simulink model "controller1"  (Simulink 7.6)
settings: Solver=ode45  StartTime=0.0  StopTime=te  MinStep=1e-9  RelTol=1e-3
undefined symbols (not defined in the file): K, traj
libraries: commnoisgen2 x4, simulink_extras x1
settings Model: Creator=tarik  LastModifiedBy=tarik

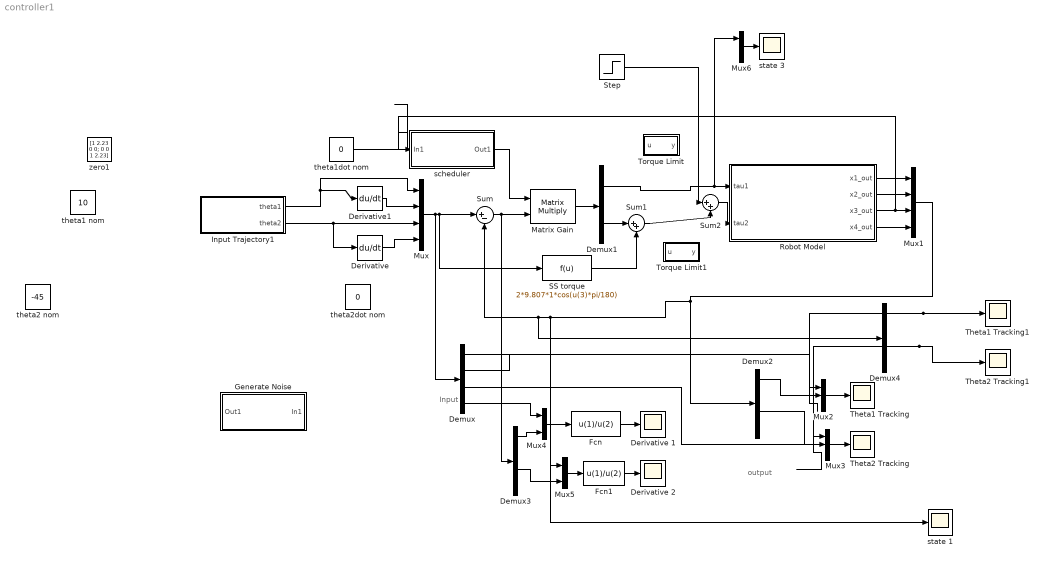
== system controller1 ==
  note: Input
  note: output
  Demux{,2..4} (4 alike) : Demux
  Demux1 : Demux  Outputs=2
  Derivative : Derivative
  Derivative 1 : Scope
      settings: TimeRange=0.09  YMin=0  YMax=70  SaveName=ScopeData3
  Derivative 2 : Scope
      settings: TimeRange=0.09  YMin=0  YMax=70  SaveName=ScopeData4
  Derivative1 : Derivative
  Fcn : Fcn  Expr=u(1)/u(2)
  Fcn1 : Fcn  Expr=u(1)/u(2)
  Generate Noise : Subsystem
  Input Trajectory1 : Subsystem
  Matrix Gain : Product  Multiplication=Matrix(*)
  Mux : Mux
  Mux1 : Mux
  Mux2 : Mux  Inputs=3
  Mux3 : Mux  Inputs=3
  Mux4 : Mux  Inputs=2
  Mux5 : Mux  Inputs=2
  Mux6 : Mux  Inputs=2
  Robot Model : Subsystem
  SS torque : Fcn  Expr=2*9.807*1*cos(u(3)*pi/180)
  Step : Step  Time=3  After=0  SampleTime=0
  Sum : Sum  Inputs=|+-
  Sum1 : Sum  Inputs=|++
  Sum2 : Sum  Inputs=|++
  Theta1 Tracking : Scope
      settings: TimeRange=0.09  YMin=-120  YMax=30
  Theta1 Tracking1 : Scope
      settings: TimeRange=0.09  YMin=-171  YMax=-163.5  SaveName=ScopeData5
  Theta2 Tracking : Scope
      settings: TimeRange=0.09  YMin=-90  YMax=-25
  Theta2 Tracking1 : Scope
      settings: TimeRange=0.09  YMin=-90  YMax=-25  SaveName=ScopeData6
  Torque Limit : Stateflow chart  TreatAsAtomicUnit=on
  Torque Limit1 : Stateflow chart  TreatAsAtomicUnit=on
  scheduler : Subsystem
  state 1 : Scope
      settings: TimeRange=0.09  YMin=-180  YMax=30  SaveName=ScopeData7
  state 3 : Scope
      settings: TimeRange=0.09  YMin=-80  YMax=80  SaveName=ScopeData2
  theta1 nom : Constant  Value=10
  theta1dot nom : Constant  Value=0
  theta2 nom : Constant  Value=-45
  theta2dot nom : Constant  Value=0
  zero1 : Constant  Value=[1 2.23 0 0; 0 0 1 2.23]
  wires:
  Mux/1 -> Demux/1, Sum/1, SS torque/1
  Robot Model/1(x1_out) -> Mux1/1
  Robot Model/2(x2_out) -> Mux1/2
  Robot Model/4(x4_out) -> Mux1/4
  Mux1/1 -> Demux2/1, Sum/2, Demux4/1, state 1/1
  Sum1/1 -> Sum2/2
  SS torque/1 -> Sum1/2
  Matrix Gain/1 -> Demux1/1
  Demux1/2 -> Sum1/1
  Sum/1 -> Matrix Gain/2, Demux3/1
  Demux1/1 -> Robot Model/1(tau1), Mux6/1
  Input Trajectory1/1(theta1) -> Mux/1, Derivative1/1
  Demux2/1 -> Mux2/2
  Mux2/1 -> Theta1 Tracking/1
  Mux3/1 -> Theta2 Tracking/1
  scheduler/1(Out1) -> Matrix Gain/1
  Input Trajectory1/2(theta2) -> Mux/3, Derivative/1
  Demux/3 -> Mux3/1
  Demux2/3 -> Mux3/2
  Derivative1/1 -> Mux/2
  Derivative/1 -> Mux/4
  Mux4/1 -> Fcn/1
  Demux/2 -> Mux5/1
  Demux/4 -> Mux4/1
  Demux3/1 -> Mux4/2
  Demux3/3 -> Mux5/2
  Mux5/1 -> Fcn1/1
  Fcn1/1 -> Derivative 2/1
  Fcn/1 -> Derivative 1/1
  Demux/1 -> Mux2/1
  Robot Model/3(x3_out) -> Mux1/3
  Mux6/1 -> state 3/1
  Sum2/1 -> Robot Model/2(tau2)
  Step/1 -> Sum2/1
  Demux4/1 -> Theta1 Tracking1/1
  Demux4/3 -> Theta2 Tracking1/1
  theta1dot nom/1 -> scheduler/1(In1)

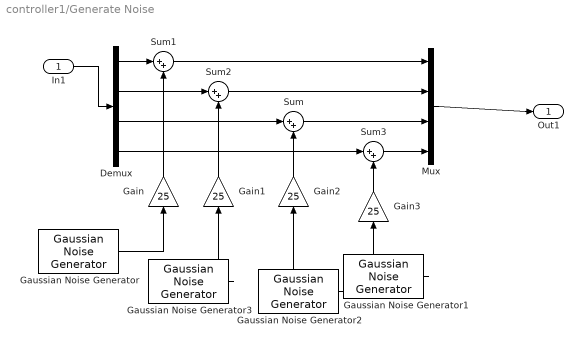
== system controller1/Generate Noise ==
  In1 : Inport
  Demux : Demux
  Gain{,1..3} (4 alike) : Gain  Gain=25
  Gaussian Noise Generator : commnoisgen2/Gaussian Noise Generator  SystemSampleTime=-1  m=0  d=1  s=41  Ts=0.1  frameBased=off  sampPerFrame=1  orient=off  outDataType=double
  Gaussian Noise Generator1 : commnoisgen2/Gaussian Noise Generator  SystemSampleTime=-1  m=0  d=1  s=41  Ts=0.1  frameBased=off  sampPerFrame=1  orient=off  outDataType=double
  Gaussian Noise Generator2 : commnoisgen2/Gaussian Noise Generator  SystemSampleTime=-1  m=0  d=1  s=41  Ts=.1  frameBased=off  sampPerFrame=1  orient=off  outDataType=double
  Gaussian Noise Generator3 : commnoisgen2/Gaussian Noise Generator  SystemSampleTime=-1  m=0  d=1  s=41  Ts=0.1  frameBased=off  sampPerFrame=1  orient=off  outDataType=double
  Mux : Mux
  Sum{,1..3} (4 alike) : Sum  Inputs=|++
  Out1 : Outport
  wires:
  In1/1 -> Demux/1
  Mux/1 -> Out1/1
  Demux/1 -> Sum1/1
  Demux/2 -> Sum2/1
  Demux/3 -> Sum/1
  Demux/4 -> Sum3/1
  Gaussian Noise Generator1/1 -> Gain3/1
  Gaussian Noise Generator2/1 -> Gain2/1
  Gaussian Noise Generator3/1 -> Gain1/1
  Gaussian Noise Generator/1 -> Gain/1
  Sum1/1 -> Mux/1
  Sum2/1 -> Mux/2
  Sum/1 -> Mux/3
  Sum3/1 -> Mux/4
  Gain/1 -> Sum1/2
  Gain1/1 -> Sum2/2
  Gain2/1 -> Sum/2
  Gain3/1 -> Sum3/2

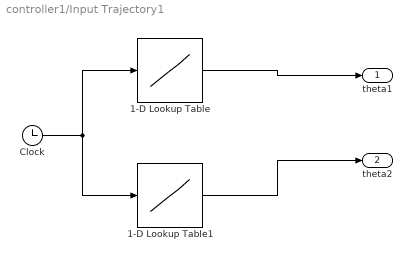
== system controller1/Input Trajectory1 ==
  1-D Lookup Table : Lookup_n-D  NumberOfTableDimensions=1  BreakpointsForDimension1=t  Table=traj(1,:)  RndMeth=Simplest  InputSameDT=on
  1-D Lookup Table1 : Lookup_n-D  NumberOfTableDimensions=1  BreakpointsForDimension1=t  Table=traj(2,:)  RndMeth=Simplest  InputSameDT=on
  Clock : Clock
      settings: Decimation=10
  theta1 : Outport
  theta2 : Outport  Port=2
  wires:
  Clock/1 -> 1-D Lookup Table/1, 1-D Lookup Table1/1
  1-D Lookup Table/1 -> theta1/1
  1-D Lookup Table1/1 -> theta2/1

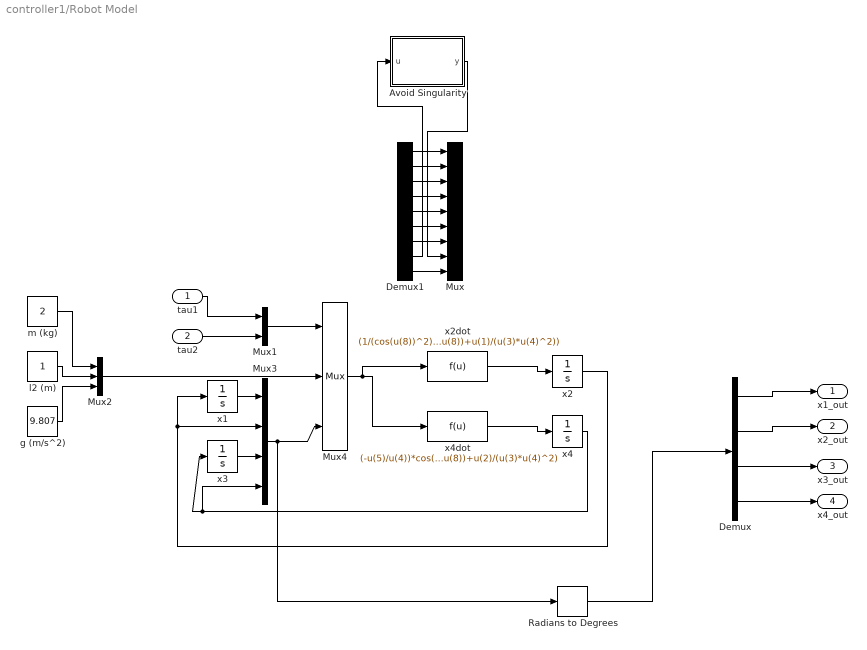
== system controller1/Robot Model ==
  tau1 : Inport
  tau2 : Inport  Port=2
  Avoid Singularity : Stateflow chart  TreatAsAtomicUnit=on
  Demux : Demux
  Demux1 : Demux  Outputs=9
  Mux : Mux  Inputs=9
  Mux1 : Mux  Inputs=2
  Mux2 : Mux  Inputs=3
  Mux3 : Mux
  Mux4 : Mux  Description=|  Inputs=3
      | u(1:2) are u1 and u2   
      | u(3:5) are m, l2, and g
      | u(6:9) are x1 x2 x3 x4
  Radians to Degrees : simulink_extras/Transformations/Radians to Degrees  SystemSampleTime=-1
  g (m/s^2) : Constant  Value=9.807
  l2 (m) : Constant
  m (kg) : Constant  Value=2
  x1 : Integrator
  x2 : Integrator
  x2dot : Fcn  Expr=(1/(cos(u(8))^2))*(u(7)*u(9)*sin(2*u(8))+u(1)/(u(3)*u(4)^2))
  x3 : Integrator  InitialCondition=0*pi/180
  x4 : Integrator
  x4dot : Fcn  Expr=(-u(5)/u(4))*cos(u(8))-(u(7)/2)*sin(2*u(8))+u(2)/(u(3)*u(4)^2)
  x1_out : Outport
  x2_out : Outport  Port=2
  x3_out : Outport  Port=3
  x4_out : Outport  Port=4
  wires:
  m (kg)/1 -> Mux2/1
  l2 (m)/1 -> Mux2/2
  g (m/s^2)/1 -> Mux2/3
  x2dot/1 -> x2/1
  x4dot/1 -> x4/1
  Mux3/1 -> Mux4/3, Radians to Degrees/1
  Mux1/1 -> Mux4/1
  x3/1 -> Mux3/3
  x4/1 -> Mux3/4, x3/1
  Mux4/1 -> x4dot/1, x2dot/1
  x2/1 -> Mux3/2, x1/1
  x1/1 -> Mux3/1
  Demux/1 -> x1_out/1
  Demux/2 -> x2_out/1
  Demux/3 -> x3_out/1
  Demux/4 -> x4_out/1
  Radians to Degrees/1 -> Demux/1
  tau1/1 -> Mux1/1
  tau2/1 -> Mux1/2
  Mux2/1 -> Mux4/2
  Demux1/1 -> Mux/1
  Demux1/2 -> Mux/2
  Demux1/3 -> Mux/3
  Demux1/4 -> Mux/4
  Demux1/5 -> Mux/5
  Demux1/6 -> Mux/6
  Demux1/7 -> Mux/7
  Demux1/9 -> Mux/9
  Demux1/8 -> Avoid Singularity/1(u)
  Avoid Singularity/1(y) -> Mux/8

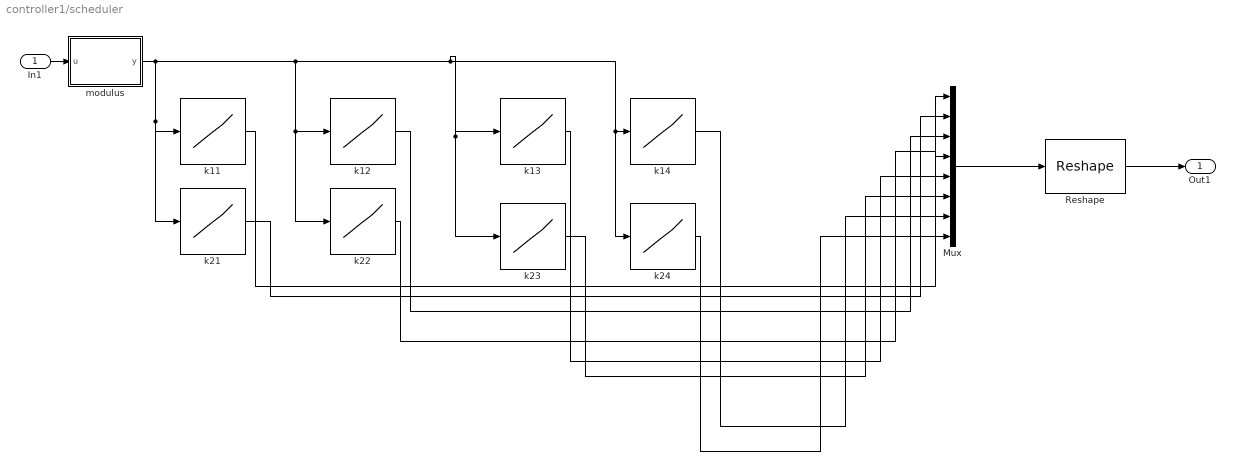
== system controller1/scheduler ==
  In1 : Inport
  Mux : Mux  Inputs=8
  Reshape : Reshape  OutputDimensionality=Customize  OutputDimensions=[2,4]
  k11 : Lookup_n-D  NumberOfTableDimensions=1  BreakpointsForDimension1=[-90:5:90]  Table=K(1,:)  RndMeth=Simplest  InputSameDT=on
  k12 : Lookup_n-D  NumberOfTableDimensions=1  BreakpointsForDimension1=[-90:5:90]  Table=K(3,:)  RndMeth=Simplest  InputSameDT=on
  k13 : Lookup_n-D  NumberOfTableDimensions=1  BreakpointsForDimension1=[-90:5:90]  Table=K(5,:)  RndMeth=Simplest  InputSameDT=on
  k14 : Lookup_n-D  NumberOfTableDimensions=1  BreakpointsForDimension1=[-90:5:90]  Table=K(7,:)  RndMeth=Simplest  InputSameDT=on
  k21 : Lookup_n-D  NumberOfTableDimensions=1  BreakpointsForDimension1=[-90:5:90]  Table=K(2,:)  RndMeth=Simplest  InputSameDT=on
  k22 : Lookup_n-D  NumberOfTableDimensions=1  BreakpointsForDimension1=[-90:5:90]  Table=K(4,:)  RndMeth=Simplest  InputSameDT=on
  k23 : Lookup_n-D  NumberOfTableDimensions=1  BreakpointsForDimension1=[-90:5:90]  Table=K(6,:)  RndMeth=Simplest  InputSameDT=on
  k24 : Lookup_n-D  NumberOfTableDimensions=1  BreakpointsForDimension1=[-90:5:90]  Table=K(8,:)  RndMeth=Simplest  InputSameDT=on
  modulus : Stateflow chart  TreatAsAtomicUnit=on
  Out1 : Outport
  wires:
  In1/1 -> modulus/1(u)
  Reshape/1 -> Out1/1
  Mux/1 -> Reshape/1
  k11/1 -> Mux/1
  k21/1 -> Mux/2
  k12/1 -> Mux/3
  k22/1 -> Mux/4
  k13/1 -> Mux/5
  k23/1 -> Mux/6
  k14/1 -> Mux/7
  k24/1 -> Mux/8
  modulus/1(y) -> k24/1, k14/1, k23/1, k13/1, k22/1, k12/1, k21/1, k11/1

== matlab function Robot Model/Avoid Singularity ==
  data: u input double; y output double
function y = fcn(u)
    th = 0.1;
    if(abs(u) > 90-th && abs(u) < 90)
        u = (90-th)*abs(u)/u;
    elseif(abs(u) > 90 && abs(u) < 90+th)
        u = (90+th)*abs(u)/u;
    end
y = u;

== matlab function scheduler/modulus ==
  data: u input double; y output double
function y = fcn(u)
    if(abs(u)>90)
        u = mod(u,90);
    end
y = u;

== matlab function Torque Limit ==
  data: u input double; y output double
% hard limit cutoff function.

function y = fcn(u)
    T = 100;
    if(abs(u) > T)
        u = T*abs(u)/u;
    end
y = u;

== matlab function Torque Limit1 ==
  data: u input double; y output double
% hard limit cutoff function.

function y = fcn(u)
    T = 100;
    if(abs(u) > T)
        u = T*abs(u)/u;
    end
y = u;
